simulink model "test"  (R2022b)
settings: Solver=VariableStepAuto  StartTime=0.0  StopTime=10.0  RelTol=1e-3
libraries: VACLib x2
settings Model: Creator=KarlO  LastModifiedBy=KarlO

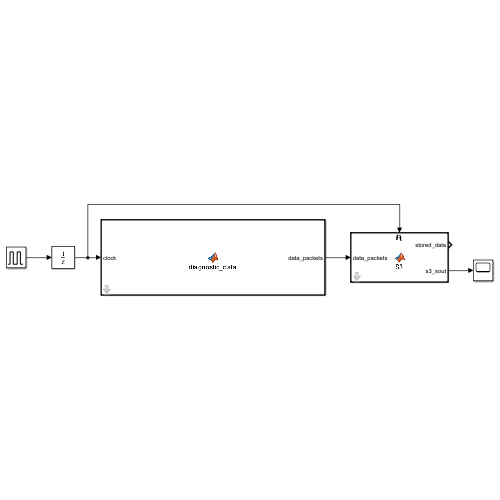
[thumbnail: Simulink's stored preview of the top-level diagram]
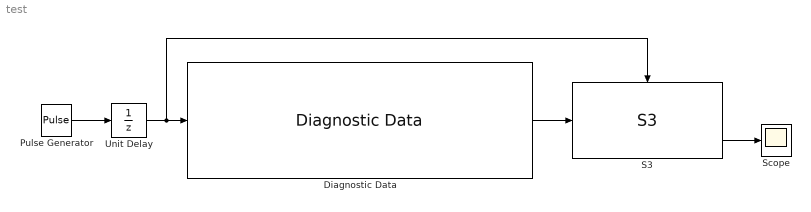
== system test ==
  Diagnostic Data : VACLib/Vehicle Components/Diagnostic Data  cache_size=32  total_data_size=20480
      settings: LibrarySourceBlock=|
      | simulink/User-Defined
      | Functions/MATLAB Function
  Pulse Generator : DiscretePulseGenerator  PulseType=Time based  PulseWidth=50
  S3 : VACLib/AWS Components/S3
      settings: LibrarySourceBlock=|
      | simulink/User-Defined
      | Functions/MATLAB Function
  Scope : Scope
  Unit Delay : UnitDelay  SampleTime=-1  HasFrameUpgradeWarning=on
  wires:
  Unit Delay/1 -> S3/Trigger, Diagnostic Data/1
  Pulse Generator/1 -> Unit Delay/1
  Diagnostic Data/1 -> S3/1
  S3/2 -> Scope/1
